simulink model "LED_RED_TEST2"  (R2020a)
settings: Solver=FixedStepAuto  StartTime=0.0  StopTime=10.0  FixedStep=1e-3  RelTol=1e-3  EnableMultiTasking=on
libraries: frdmk64flib x3, etargetslib x2
settings Model: ExtModeTrigDuration=5  Creator=jeffl  LastModifiedBy=jeffl
settings OptimizationCC: EnhancedBackFolding=on  PassReuseOutputArgsAs=Individual arguments  ZeroExternalMemoryAtStartup=off  ZeroInternalMemoryAtStartup=off  MaxStackSize=64  OptimizeBlockOrder=speed  DifferentSizesBufferReuse=on  OptimizationCustomize=off  EfficientTunableParamExpr=on
settings DebuggingCC: ParameterTunabilityLossMsg=error
settings HardwareCC: ProdBitPerPointer=32  ProdBitPerSizeT=32  ProdBitPerPtrDiffT=32  ProdLargestAtomicInteger=Long  ProdLargestAtomicFloat=Double  ProdWordSize=32  ProdHWDeviceType=ARM Compatible->ARM Cortex
settings SFSimCC: MATLABDynamicMemAlloc=off
settings RTWCC: SystemTargetFile=ert.tlc  HardwareBoard=NXP FRDM-K64F  TemplateMakefile=ert_default_tmf  Toolchain=GNU Tools for ARM Embedded Processors
settings CodeAppCC: ForceParamTrailComments=on  IgnoreCustomStorageClasses=off  OperatorAnnotations=on  SimulinkDataObjDesc=on  SFDataObjDesc=on  InsertBlockDesc=on

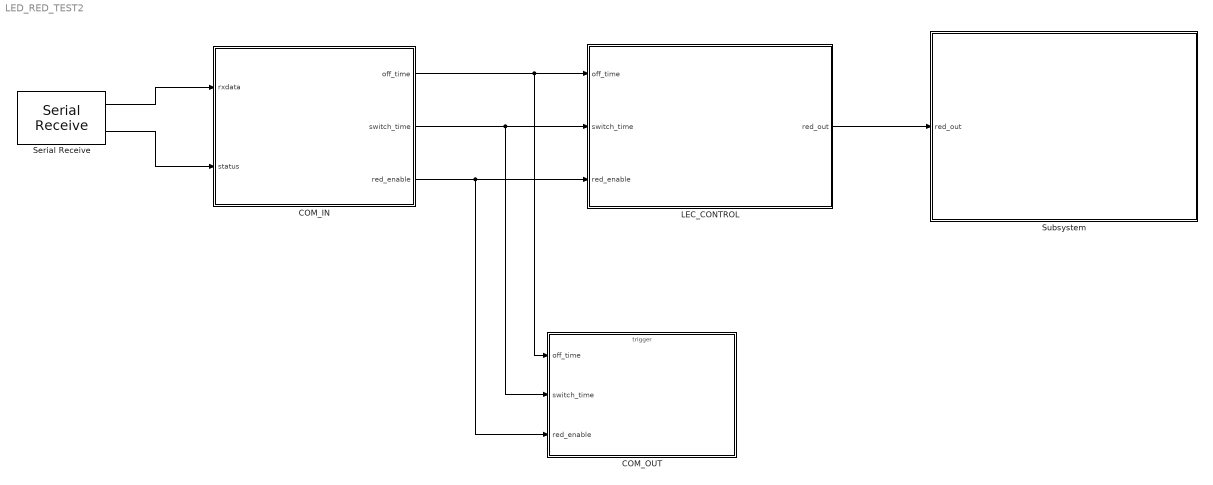
== system LED_RED_TEST2 ==
  COM_IN : Stateflow chart  TreatAsAtomicUnit=on
  COM_OUT : Subsystem  TreatAsAtomicUnit=on
  LEC_CONTROL : Stateflow chart  TreatAsAtomicUnit=on
  Serial Receive : frdmk64flib/Serial Receive  SCIModule=0  Baudrate=uint32(9600)  Parity=None  StopBits=1  HardwareFlowControl=None  ByteOrder=LittleEndian  DataType=uint8  DataLength=10  BlockingMode=off  OutputStatus=on  SampleTime=-1
  Subsystem : Subsystem
  wires:
  Serial Receive/1 -> COM_IN/1(rxdata)
  Serial Receive/2 -> COM_IN/2(status)
  COM_IN/1(off_time) -> COM_OUT/1(off_time), LEC_CONTROL/1(off_time)
  COM_IN/2(switch_time) -> COM_OUT/2(switch_time), LEC_CONTROL/2(switch_time)
  COM_IN/3(red_enable) -> COM_OUT/3(red_enable), LEC_CONTROL/3(red_enable)
  LEC_CONTROL/1(red_out) -> Subsystem/1(red_out)

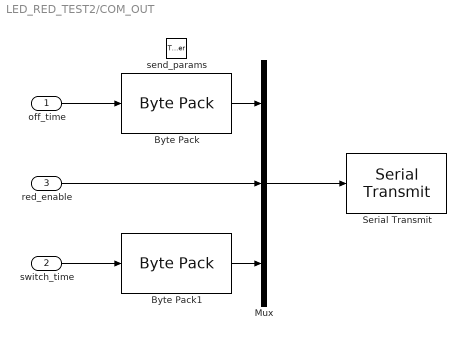
== system LED_RED_TEST2/COM_OUT ==
  off_time : Inport
  switch_time : Inport  Port=2
  red_enable : Inport  Port=3
  send_params : TriggerPort  TriggerType=function-call  IsSimulinkFunction=on  FunctionName=send_params  VariantControl=(inherit)
  Byte Pack : etargetslib/Byte Pack  datatypes={'single'}  byteAlign=1
  Byte Pack1 : etargetslib/Byte Pack  datatypes={'uint16'}  byteAlign=1
  Mux : Mux  Inputs=3
  Serial Transmit : frdmk64flib/Serial Transmit  SCIModule=0  Baudrate=uint32(9600)  Parity=None  StopBits=1  HardwareFlowControl=None  ByteOrder=LittleEndian  BlockingMode=on  OutputStatus=off
  wires:
  off_time/1 -> Byte Pack/1
  red_enable/1 -> Mux/2
  switch_time/1 -> Byte Pack1/1
  Mux/1 -> Serial Transmit/1
  Byte Pack/1 -> Mux/1
  Byte Pack1/1 -> Mux/3

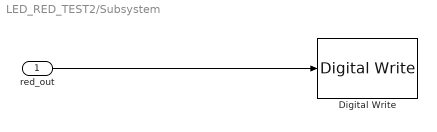
== system LED_RED_TEST2/Subsystem ==
  red_out : Inport
  Digital Write : frdmk64flib/Digital Write  Whichpin=RED_LED
  wires:
  red_out/1 -> Digital Write/1

== stateflow chart LED_RED_TEST2/LEC_CONTROL ==
  state OFF
    entry:
    red_out=0;
  state RED_ON
    entry:
    red_out=1;
  (default) -> OFF
  OFF -> (junction 8) : after(off_time,sec)
  (junction 8) -> RED_ON : [red_enable==1]
  RED_ON -> OFF : after(switch_time,msec)
  data: off_time input; switch_time input; red_enable input; red_out output

== stateflow chart LED_RED_TEST2/COM_IN ==
  settings: executeAtInitialization=1
  state SET_PARAM
    entry:
    red_enable = rxdata(3); %maybe not 3,
    off_time = typecast(rxdata(6:9),'single');%maybe not 6 to 9
    switch_time = typecast(rxdata(10:11),'uint16');
  state INITIAL
    entry:
    red_enable = 0;
    off_time =0.5; % seconds
    switch_time = 200; % in msec
  state STANDBY
  state ECHO_PARAM
    entry:
    send_params();
  SET_PARAM -> STANDBY
  (junction 12) -> SET_PARAM [order 1] : [rxdata(2) == hex2dec('55')]
  (default) -> INITIAL
  (junction 11) -> STANDBY [order 2]
  INITIAL -> STANDBY
  STANDBY -> (junction 11) : [status == 0]
  (junction 11) -> (junction 12) [order 1] : [rxdata(1) == hex2dec('16')]
  (junction 12) -> ECHO_PARAM [order 2] : [rxdata(2) == hex2dec('22')]
  ECHO_PARAM -> STANDBY
  data: rxdata input uint8; status input boolean; off_time output single; switch_time output uint16; red_enable output uint8
